simulink model "refMag"  (R2018a)
settings: Solver=VariableStepAuto  StartTime=0.0  StopTime=10.0  RelTol=1e-3
settings Model: Creator=nathan  LastModifiedBy=nathan

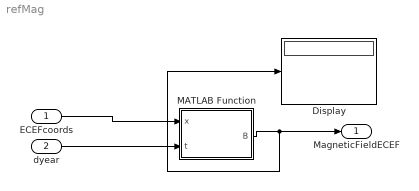
== system refMag ==
  ECEFcoords : Inport  Unit=m
  dyear : Inport  Port=2
  Display : Display
  MATLAB Function : MATLAB Function  TreatAsAtomicUnit=on
  MagneticFieldECEF : Outport  Unit=G
  wires:
  MATLAB Function/1(B) -> Display/1, MagneticFieldECEF/1
  ECEFcoords/1 -> MATLAB Function/1(x)
  dyear/1 -> MATLAB Function/2(t)

== matlab function refMag/MATLAB Function ==
  data: x input; B output; t input
function B = fcn(x,t)
% fnc runs geomag c function in '../libraries/GeoMag.c' and returns the
% feild, units gauss ECEF
B=zeros([3,1]);

coder.updateBuildInfo('addSourceFiles','GeoMag.c');
coder.cinclude('GeoMag.h');

xstruct= struct('x',x(1),'y',x(2),'z',x(3));
coder.cstructname(xstruct,'MAGtype_CoordECEF','extern','HeaderFile','GeoMag.h');
rstruct= struct('Bx',B(1),'By',B(2),'Bz',B(3));
coder.cstructname(rstruct,'MAGtype_MagneticResults','extern','HeaderFile','GeoMag.h');
coder.ceval('MAG_geomag',xstruct,t,coder.ref(rstruct));
B(1)= rstruct.Bx;
B(2)= rstruct.By;
B(3)= rstruct.Bz;
